simulink model "First_Model_2026_SIMULATION_ONLY_FINAL"  (R2022b)
settings: Solver=VariableStepAuto  StartTime=0.0  StopTime=50  RelTol=1e-3
model workspace (MAT data in the model file):
  dt = 0.01
libraries: simulink x3
(part 2 of 2)

== matlab function First_Model_2026_SIMULATION_ONLY_FINAL/UKF_algorithm/UKF_Static ==
  data: x_i input; y_i input; beta_i input; est_x output; est_y output; exec_time output
function [est_x, est_y, exec_time] = UKF_Static(x_i, y_i, beta_i)
    % UKF_Static_Final
    % Unscented Kalman Filter for Static Target (6-State).
    % Estimates: [Target_X, Target_Y, Self_X, Self_Vx, Self_Y, Self_Vy]
    
    persistent X_est P Q R 
    
    % --- Timing ---
    exec_time = 0; 
    coder.extrinsic('tic', 'toc'); 
    tStart = tic; 
    
    % --- Initialization ---
    if isempty(P)
        nx = 6; % State Dimension
        
        % 1. Covariance (P) - High uncertainty
        P = 1000 * eye(nx); 
        
        % 2. Process Noise (Q)

        Q = 0.001 * diag([0.01, 0.01, 100, 10, 100, 10]); 
        
        % 3. Measurement Noise (R)
        % [Self_X, Self_Y, Constraint]
        % UPDATED: Matches your Simulink noise (5) and Constraint (200)
        R = diag([5, 5, 200]); 
    end
    
    if isempty(X_est)
        X_est = zeros(6, 1); 
    end
    
    % --- UKF Parameters (Calculated every step, like student code) ---
    nx = 6;
    alpha = 1e-3; 
    beta_param = 2; 
    kappa = 0; 
    lambda = alpha^2 * (nx + kappa) - nx;
    
    % Weights
    Wm = [lambda / (nx + lambda); repmat(1 / (2 * (nx + lambda)), 2 * nx, 1)];
    Wc = Wm;
    Wc(1) = Wc(1) + (1 - alpha^2 + beta_param);
    
    dt = 0.01; % Sample time
    
    % ===========================================
    % 1. GENERATE SIGMA POINTS
    % ===========================================
    
    % FIX: Diagonal Loading (Replaces try/catch)
    % Ensures P is Positive Definite so chol() never crashes
    P_stable = P + 1e-9 * eye(nx);
    
    S = chol((nx + lambda) * P_stable, 'lower');
    sigma_points = [X_est, bsxfun(@plus, X_est, S), bsxfun(@minus, X_est, S)];
    
    % ===========================================
    % 2. PREDICT STEP (Time Update)
    % ===========================================
    
    % Pass through Static Process Model (Target V=0)
    predicted_sigmas = process_model_static(sigma_points, dt);
    
    % Recover Mean and Covariance
    [X_pred, P_pred] = compute_mean_and_cov(predicted_sigmas, Wm, Wc, Q);
    
    % ===========================================
    % 3. UPDATE STEP (Measurement Update)
    % ===========================================
    
    % Pass through Pseudolinear Measurement Model
    measured_sigmas = measurement_model(predicted_sigmas, beta_i);
    
    % Recover Measurement Mean and Covariance
    [y_pred, Pyy] = compute_mean_and_cov(measured_sigmas, Wm, Wc, R);
    
    % Cross-Covariance
    Pxy = compute_cross_cov(predicted_sigmas, measured_sigmas, X_pred, y_pred, Wc);
    
    % Kalman Gain
    K = Pxy / Pyy;
    
    % Measurement Vector (Observed)
    z_meas = [x_i; y_i; 0]; 
    
    % Update State and Covariance
    resid = z_meas - y_pred;
    X_est = X_pred + K * resid;
    P = P_pred - K * Pyy * K';
    
    % SAFETY: Force Symmetry
    P = 0.5 * (P + P');
    
    % --- Outputs ---
    est_x = X_est(1); % Target X
    est_y = X_est(2); % Target Y
    
    exec_time = toc(tStart); 
end

%% --- Helper Functions ---

function points_out = process_model_static(points_in, dt)
    % Static Model: Target Velocity is 0. Self Velocity is constant.
    % 6x6 Matrix
    F = [1 0 0 0 0 0;  % Tx
         0 1 0 0 0 0;  % Ty
         0 0 1 dt 0 0; % Sx
         0 0 0 1 0 0;  % Svx
         0 0 0 0 1 dt; % Sy
         0 0 0 0 0 1]; % Svy
         
    points_out = F * points_in;
end

function points_out = measurement_model(points_in, beta)
    % Pseudolinear Measurement Matrix
    s = sin(beta);
    c = cos(beta);
    
    % H Matrix (3x6)
    % Rows 1-2: Measure Self X (Idx 3) and Self Y (Idx 5)
    % Row 3: Constraint involving Tx(1), Ty(2), Sx(3), Sy(5)
    H = [0 0 1 0 0 0;    % Self X
         0 0 0 0 1 0;    % Self Y
         s, -c, -s, 0, c, 0]; % Constraint
         
    points_out = H * points_in;
end

function [mean_out, cov_out] = compute_mean_and_cov(sigmas, Wm, Wc, NoiseCov)
    % Weighted Mean
    mean_out = sigmas * Wm;
    
    % Weighted Covariance
    d = bsxfun(@minus, sigmas, mean_out);
    cov_out = d * diag(Wc) * d' + NoiseCov;
end

function Pxy = compute_cross_cov(sig_pred, sig_meas, x_mean, y_mean, Wc)
    % Cross Covariance
    dx = bsxfun(@minus, sig_pred, x_mean);
    dy = bsxfun(@minus, sig_meas, y_mean);
    Pxy = dx * diag(Wc) * dy';
end

== matlab function First_Model_2026_SIMULATION_ONLY_FINAL/errors_and_display_ukf/Calculate_axis_ukf ==
  data: x_est input; pct_err_x output; y_est input; x_tgt input; y_tgt input; pct_err_y output; sleeve_x_up output; sleeve_x_down output; sleeve_y_up output; sleeve_y_down output
function [pct_err_x, pct_err_y, sleeve_x_up, sleeve_x_down, sleeve_y_up, sleeve_y_down] = Calculate_axis_errors(x_est, y_est, x_tgt, y_tgt)
    % Inputs:
    %   x_est, y_est: Estimated position
    %   x_tgt, y_tgt: Real Target position

    % --- 1. Calculate Percentage Errors (Per Axis) ---
    % Useful for statistics: "What is my % error on X?"
    if abs(x_tgt) < 0.001, x_tgt = 0.001; end
    if abs(y_tgt) < 0.001, y_tgt = 0.001; end
    
    pct_err_x = ((x_est - x_tgt) / x_tgt) * 100;
    pct_err_y = ((y_est - y_tgt) / y_tgt) * 100;

    % --- 2. Calculate Sleeve Bounds (The "Tunnel") ---
    % Useful for Visualization: Plot 'x_est' against these two lines.
    
    % Calculate 10% margin based on absolute position
    margin_x = 0.1 * abs(x_tgt);
    margin_y = 0.1 * abs(y_tgt);
    
    % Define Upper and Lower walls of the tunnel
    sleeve_x_up   = x_tgt + margin_x; % Real X + 10%
    sleeve_x_down = x_tgt - margin_x; % Real X - 10%
    
    sleeve_y_up   = y_tgt + margin_y; % Real Y + 10%
    sleeve_y_down = y_tgt - margin_y; % Real Y - 10%
end

== matlab function First_Model_2026_SIMULATION_ONLY_FINAL/errors_and_display_ukf/Distance _error_ukf ==
  data: x_est input; y_est input; pct_err_dist output; x_tgt input; y_tgt input; ref_plus_10 output; ref_minus_10 output
function [pct_err_dist, ref_plus_10, ref_minus_10] = Distance_error_ukf(x_est, y_est, x_tgt, y_tgt)
    % Inputs:
    %   x_est, y_est: Estimated position (from EKF)
    %   x_tgt, y_tgt: Real Target position
    
    % --- 1. Calculate Distances (Range) ---
    dist_est = sqrt(x_est^2 + y_est^2);
    dist_tgt = sqrt(x_tgt^2 + y_tgt^2);
    
    % Safety for division by zero
    if dist_tgt < 0.001
        dist_tgt = 0.001;
    end

    % --- 2. Calculate Percentage Error ---

    pos_err = sqrt((x_est - x_tgt)^2 + (y_est - y_tgt)^2);

    pct_err_dist = (pos_err / dist_tgt) * 100;
    
    % --- 3. Reference Lines (Constants) ---
    % Since the output is Percentage, the bounds are simply +10 and -10.
    ref_plus_10 = 10;
    ref_minus_10 = -10;
end

== matlab function First_Model_2026_SIMULATION_ONLY_FINAL/Observer_Position/Linear_transformation ==
  data: x_init input; y_init input; v_x input; v_y input; t input; x_linear output; y_linear output
function [x_linear, y_linear] = Kinematics_Linear(x_init, y_init, v_x, v_y, t)
    % Kinematics_Linear Calculates self position for a constant velocity path.
    %
    % Inputs: 
    %   x_init, y_init: Initial position (meters)
    %   v_x, v_y: Constant velocities (m/s)
    %   t: Current simulation time (seconds)
    
    % --- Linear Motion (ENU Coordinates) ---
    % Standard kinematic equation: position = initial_position + velocity * time
    x_linear = x_init + v_x * t;
    y_linear = y_init + v_y * t;

== matlab function First_Model_2026_SIMULATION_ONLY_FINAL/Observer_Position/Lemniscate_transformation ==
  data: x_init input; y_init input; t input; w input; x_lemniscate output; y_lemniscate output; a input
function [x_lemniscate, y_lemniscate] = Kinematics_Lemniscate(x_init, y_init, t, w, a)
    % Kinematics_Circular_and_Lemniscate Calculates self position for circular and lemniscate paths.
    % These complex paths ensure the required 'excitation' for passive tracking observability.
    %
    % Inputs: 
    %   x_init, y_init: Initial position (meters). Used for center offset and radius/width calculation.
    %   t: Current simulation time (seconds).
    %   w: Angular velocity (rad/s), controls the speed of the motion.
    
    % --- 1. Calculate Radius/Width (R) ---
    % R is determined by the distance from the origin (0,0) to the initial position (x_init, y_init).
    R = sqrt(x_init^2 + y_init^2);
    
    % Safety check: If starting at (0,0), set a minimum radius/width to ensure movement.
    if R == 0
        R = 100; % Default to a 100m scale.
    end

    
    % --- 3. Lemniscate (Figure-8) Motion (Outputs: x_lemniscate, y_lemniscate) ---
    % Lemniscate of Bernoulli equations: x = a*cos(theta)/denom, y = a*sin(theta)*cos(theta)/denom
    % We use R as the width parameter 'a' (a_lemniscate).
    
    a_lemniscate = a * sqrt(2); 
    
    theta = w * t;
    denom = 1 + sin(theta)^2;
    
    % Calculate position relative to (0,0)
    x_local = (a_lemniscate * cos(theta)) ./ denom;
    y_local = (a_lemniscate * sin(theta) .* cos(theta)) ./ denom;
    
    % Shift the figure-8 so it is centered near the initial position
    x_lemniscate = x_local + x_init;
    y_lemniscate = y_local + y_init;

== matlab function First_Model_2026_SIMULATION_ONLY_FINAL/RLS_algorithm/RLS_Static ==
  data: x_observer input; y_observer input; beta input; x_rls output; y_rls output; exec_time output
function [x_rls, y_rls, exec_time] = RLS_Static(x_observer, y_observer, beta)
    % Inputs:
    %   x_observer, y_observer: Our ship's current position
    %   beta: Measured angle to target in radians

    persistent P X_est
    

    
    % Performance tracking
    exec_time = 0;
    coder.extrinsic('tic', 'toc');
    tStart = tic;

    % Initialization
    if isempty(P)
        P = 10000 * eye(2); % High initial uncertainty
        X_est = [0; 0];     % Initial guess (could be improved if you have a range guess)
    end

    % Pseudolinear Measurement Vector
    % Model: x_target * sin(beta) - y_target * cos(beta) = x_obs * sin(beta) - y_obs * cos(beta)
    
    sin_b = sin(beta);
    cos_b = cos(beta);

    % Measurement Matrix H
    H = [sin_b, -cos_b]; 
    
    % The "Pseudo-measurement" z
    z = x_observer * sin_b - y_observer * cos_b;

    % --- RLS Update ---
    
    % 1. Calculate Gain
    % We use R_cov here instead of '1'
    S = H * P * H' + 1; 
    K = (P * H') / S;

    % 2. Error (Innovation)
    e = z - H * X_est;

    % 3. Update State
    X_est = X_est + K * e;

    % 4. Update Covariance
    P = (eye(2) - K * H) * P;

    % --- Outputs ---
    x_rls = X_est(1);
    y_rls = X_est(2);
    exec_time = toc(tStart);
end

== matlab function First_Model_2026_SIMULATION_ONLY_FINAL/RLS_algorithm/RLS_Dynamic ==
  data: x_i input; y_i input; beta_i input; est_x output; est_y output; exec_time output
function [est_x, est_y, exec_time] = RLS_Dynamic(x_i, y_i, beta_i) 
% RLS_Dynamic_Final
% Performs Recursive Least Squares (RLS) tracking for a moving target.
% Inputs:
%
%   x_i, y_i : Our Ship's Position (Self)
%   beta_i   : Noisy Angle Measurement (Radians)
% Outputs:
%   est_x, est_y : Estimated Target Position

% --- Persistent Memory ---
persistent P X_i lambda lambda_rate

% --- Timing Setup ---
exec_time = 0; 
coder.extrinsic('tic', 'toc'); 
tStart = tic; 

% --- Initialization (Runs once at t=0) ---
if isempty(P)
    % We set P to 10000 so the filter isn't "stubborn" at the start.
    % It allows the estimate to snap to the true position in short time.
    P = 10000 * eye(2);  
    
    % FIX 2: Tuned Forgetting Factor (Lambda)
    % We start with a lower lambda to learn quickly, then slowly increase it.
    lambda = 0.95; 
    
    % The 'Rate' controls how fast it hardens. 
    lambda_rate = 0.8; 
end

if isempty(X_i)
    X_i = zeros(2, 1);  % X vector initialization as a zero vector
end

% --- 1. Construct Pseudolinear Measurement ---
% Measurement Vector (phi) and Scalar (z)
% Model: -x*sin(beta) + y*cos(beta) = y_obs*cos(beta) - x_obs*sin(beta)
phi_i = [-sin(beta_i); cos(beta_i)];
z_i   = y_i * cos(beta_i) - x_i * sin(beta_i);

% --- 2. Calculate RLS Updates ---

% A. Estimation Error
e = z_i - phi_i' * X_i;

% B. Calculate Gain Vector (g_k)
% We use 3e-5 for R (Noise Variance) to scale the denominator correctly.
R_cov = 3e-5; 
denominator = (lambda * R_cov) + (phi_i' * P * phi_i);
g_k = (P * phi_i) / denominator;

% C. Update State Vector (Position Estimate)
X_i = X_i + g_k * e;

% D. Update Covariance Matrix (P)
P = (1 / lambda) * (P - g_k * phi_i' * P);

% Prevents numerical crashes over long simulations.
P = 0.5 * (P + P');

% --- 3. Update Lambda (Annealing with Safety Cap) ---
% Slowly increase lambda to smooth out the noise...
lambda = lambda_rate * lambda + (1 - lambda_rate);

if lambda > 0.9999999
    lambda = 0.9999999;
end

% --- Outputs ---
est_x = X_i(1);
est_y = X_i(2);
exec_time = toc(tStart); 
end

== matlab function First_Model_2026_SIMULATION_ONLY_FINAL/Target_position/Calculating_different_positions/linear position ==
  data: x_i input; x_lin output; y_i input; v_x input; v_y input; t input; y_lin output
function [x_lin, y_lin] = lin_target_pos(x_i, y_i, v_x, v_y, t)
    % Calculate the linear position in the X direction
    % Formula: x(t) = x_initial + (velocity_x * time)
    x_lin = x_i + (v_x * t);

    % Calculate the linear position in the Y direction
    % Formula: y(t) = y_initial + (velocity_y * time)
    y_lin = y_i + (v_y * t);

== matlab function First_Model_2026_SIMULATION_ONLY_FINAL/Angle_Calculation ==
  data: self_pos_x input; beta output; self_pos_y input; target_pos_x input; target_pos_y input
function beta = angle_beta_calc(self_pos_x, self_pos_y, target_pos_x, target_pos_y)

% Calculate relative position (target relative to self)
dx = target_pos_x - self_pos_x;   % delta x
dy = target_pos_y - self_pos_y;   % delta y

% Line-of-sight (bearing) angle beta from self to target
% atan2 returns angle in radians, from -pi to +pi
% Positive angle is counterclockwise from the positive x-axis
beta = atan2(dy, dx);

== matlab function First_Model_2026_SIMULATION_ONLY_FINAL/Unwrapping ==
  settings: updateMethod=DISCRETE
  data: beta input; beta_unwrapped output
function beta_unwrapped = angle_unwrapper(beta)
%#codegen

% Persistent variable to store previous unwrapped angle
persistent beta_prev;
if isempty(beta_prev)
    beta_prev = 0;  % initial value on first call
end

% Define threshold for detecting 2π jumps
threshold = pi;

% Compute angle difference
delta = beta - mod(beta_prev, 2*pi);

% Unwrap: detect jumps larger than π and correct by ±2π
if delta > threshold
    delta = delta - 2*pi;
elseif delta < -threshold
    delta = delta + 2*pi;
end

% Update unwrapped angle
beta_unwrapped = beta_prev + delta;

% Save for next step
beta_prev = beta_unwrapped;

end
